simulink model "fuzz"  (R2022b)
settings: Solver=VariableStepAuto  StartTime=0.0  StopTime=10  RelTol=1e-3
libraries: fuzblock x2, vrlib x2
settings Model: Creator=philf  LastModifiedBy=philf

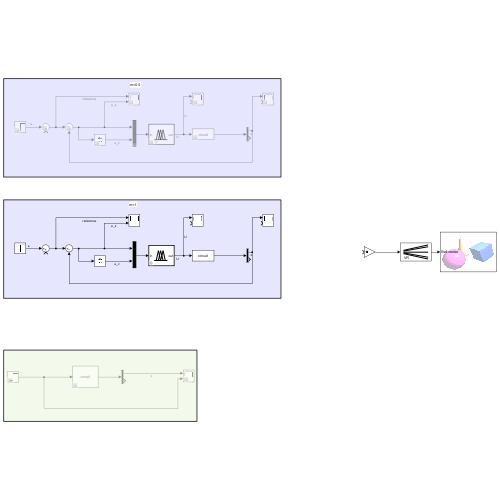
[thumbnail: Simulink's stored preview of the top-level diagram]
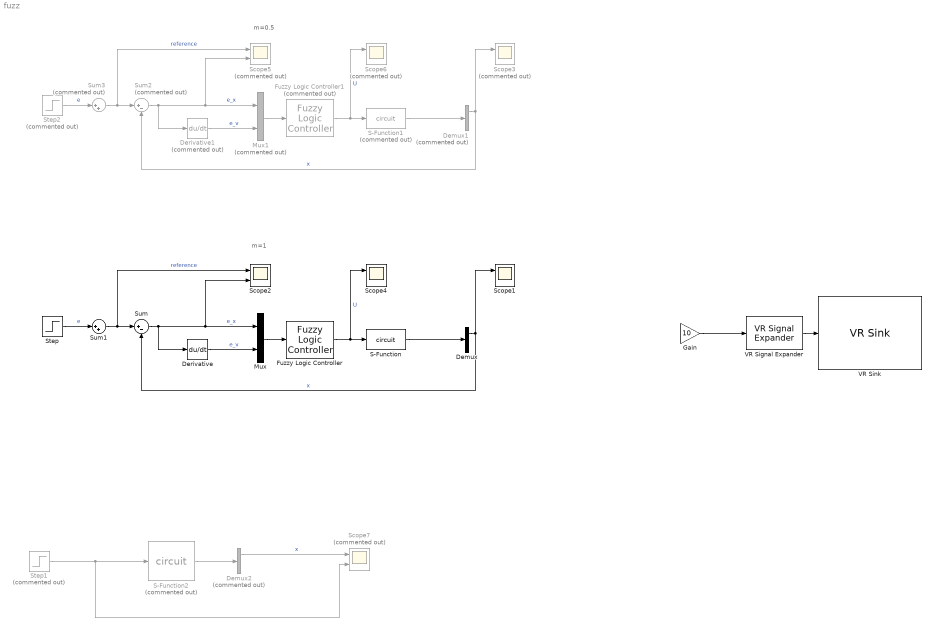
== system fuzz ==
  note: m=1
  note: m=0.5
  Demux : Demux  Outputs=2
  Demux1 : Demux  Commented=on  Outputs=2
  Demux2 : Demux  Commented=on  Outputs=2
  Derivative : Derivative
  Derivative1 : Derivative  Commented=on
  Fuzzy Logic Controller : fuzblock/Fuzzy Logic  Controller  FIS='controller_x1_2'  OutputSampleNumber=101  DataType=double  FuzzifiedInputs=off  RuleFiringStrengths=off  RuleOutputs=off  AggregatedOutputs=off  SimulateUsing=Interpreted execution  OutOfRangeInputValueMessage=warning  NoRuleFiredMessage=warning  EmptyOutputFuzzySetMessage=warning
  Fuzzy Logic Controller1 : fuzblock/Fuzzy Logic  Controller  Commented=on  FIS='controller_x1_1'  OutputSampleNumber=101  DataType=double  FuzzifiedInputs=off  RuleFiringStrengths=off  RuleOutputs=off  AggregatedOutputs=off  SimulateUsing=Interpreted execution  OutOfRangeInputValueMessage=warning  NoRuleFiredMessage=warning  EmptyOutputFuzzySetMessage=warning
  Gain : Gain  Gain=10
  Mux : Mux  Inputs=2
  Mux1 : Mux  Commented=on  Inputs=2
  S-Function : S-Function  FunctionName=circuit  Parameters=m,g,K,R,L  SFunctionDeploymentMode=off  EnableBusSupport=off  mask{m=0.1, g=9.81, K=0.005, R=5, L=0.01}
      mask prompts: R "电阻"; L "电感"
      mask DialogControl ParameterGroupVar Prompt: 参数
  S-Function1 : S-Function  Commented=on  FunctionName=circuit  Parameters=m,g,K,R,L  SFunctionDeploymentMode=off  EnableBusSupport=off  mask{m=0.5, g=9.81, K=0.005, R=5, L=0.01}
      mask prompts: R "电阻"; L "电感"
      mask DialogControl ParameterGroupVar Prompt: 参数
  S-Function2 : S-Function  Commented=on  FunctionName=circuit  Parameters=m,g,K,R,L  SFunctionDeploymentMode=off  EnableBusSupport=off  mask{m=0.05, g=9.81, K=0.005, R=5, L=0.01}
      mask prompts: R "电阻"; L "电感"
      mask DialogControl ParameterGroupVar Prompt: 参数
  Scope1 : Scope  NumInputPorts=2
  Scope2 : Scope  NumInputPorts=2
  Scope{3,5..7} (4 alike) : Scope  Commented=on  NumInputPorts=2
  Scope4 : Scope  NumInputPorts=2
  Step : Step  Time=0  After=0.05  SampleTime=0
  Step1 : Step  Commented=on  Time=0  After=10  SampleTime=0
  Step2 : Step  Commented=on  Time=0  After=0.05  SampleTime=0
  Sum : Sum  Inputs=|+-
  Sum1 : Sum  Inputs=|++
  Sum2 : Sum  Commented=on  Inputs=|+-
  Sum3 : Sum  Commented=on  Inputs=|++
  VR Signal Expander : vrlib/VR Signal Expander  outwidth=3  outidx=2
  VR Sink : vrlib/VR Sink  InstantiateOnLoad=on  SampleTime=0.1  ViewEnable=on  RemoteChange=off  RemoteView=off  FieldsWritten=Ball.center.3.1.1.double  WorldFileName=resources\bouncingball.x3d  WorldDescription=VR Bouncing Ball  AutoView=off  VideoDimensions=[]  AllowVariableSize=off
  wires:
  S-Function/1 -> Demux/1
  Mux/1 -> Fuzzy Logic Controller/1
  VR Signal Expander/1 -> VR Sink/1
  S-Function2/1 -> Demux2/1
  Step1/1 -> Scope7/2, S-Function2/1
  Demux2/1 -> Scope7/1  "x"
  Step/1 -> Sum1/1  "e"
  Demux/1 -> Sum/2, Scope1/1  "x"
  Derivative/1 -> Mux/2  "e_v"
  Sum/1 -> Mux/1, Scope2/2, Derivative/1  "e_x"
  Fuzzy Logic Controller/1 -> S-Function/1, Scope4/1  "U"
  Sum1/1 -> Scope2/1, Sum/1  "reference"
  Gain/1 -> VR Signal Expander/1
  Sum3/1 -> Scope5/1, Sum2/1  "reference"
  Demux1/1 -> Sum2/2, Scope3/1  "x"
  Fuzzy Logic Controller1/1 -> S-Function1/1, Scope6/1  "U"
  Sum2/1 -> Mux1/1, Scope5/2, Derivative1/1  "e_x"
  S-Function1/1 -> Demux1/1
  Mux1/1 -> Fuzzy Logic Controller1/1
  Derivative1/1 -> Mux1/2  "e_v"
  Step2/1 -> Sum3/1  "e"
